simulink model "simulink_group46"  (R2022b)
settings: Solver=FixedStepAuto  StartTime=0.0  StopTime=10  FixedStep=1e-3  RelTol=1e-3  EnableMultiTasking=on
undefined symbols (not defined in the file): A0, A1, D0, D1, D10, D11, D12, D13, D2, D3, D4, D5, D6, D7, D8, D9, PTA0, PTA1, PTA2, PTB2, PTB23, PTB3, PTB9, PTC16, PTC17, PTC2, PTC3, PTC4, PTD0, PTD1, PTD2, PTD3
libraries: frdmk64flib x19, etargetslib x19, dspstat3 x1
settings Model: ExtModeTrigDuration=5  Creator=aliciamorielli  LastModifiedBy=ethan
settings SolverCC: AlgebraicLoopSolver=TrustRegion
settings OptimizationCC: EnhancedBackFolding=on  PassReuseOutputArgsThreshold=0  MaxStackSize=64  OptimizeBlockOrder=speed  DifferentSizesBufferReuse=on  OptimizationCustomize=off
settings DebuggingCC: ParameterTunabilityLossMsg=error  UnconnectedInputMsg=warning  UnconnectedOutputMsg=warning  UnconnectedLineMsg=warning  SFMachineParentedDataDiag=warning
settings HardwareCC: ProdBitPerPointer=32  ProdBitPerSizeT=32  ProdBitPerPtrDiffT=32  ProdLargestAtomicInteger=Long  ProdLargestAtomicFloat=Double  ProdWordSize=32  ProdHWDeviceType=ARM Compatible->ARM Cortex  UseEmbeddedCoderFeatures=off
settings ModelReferenceCC: EnableRefExpFcnMdlSchedulingChecks=on
settings SFSimCC: MATLABDynamicMemAlloc=off
settings RTWCC: Description=Embedded Coder  SystemTargetFile=ert.tlc  HardwareBoard=NXP FRDM-K64F  TLCOptions="-aInlineSetEventsForThisBaseRateFcn=TLC_FALSE -aSuppressMultiTaskScheduler=TLC_FALSE  -aRateBasedStepFcn=0"  TemplateMakefile=ert_default_tmf  Toolchain=GNU Tools for ARM Embedded Processors  DLArmComputeVersion=19.05
settings CodeAppCC: ForceParamTrailComments=on  OperatorAnnotations=on
settings ERTTargetCC: ERTCustomFileBanners=off  SupportContinuousTime=on  SupportNonInlinedSFcns=on  RemoveResetFunc=off  ModelStepFunctionPrototypeControlCompliant=off  ExtModeTransport=4  ExtModeMexFile=sendToCommService

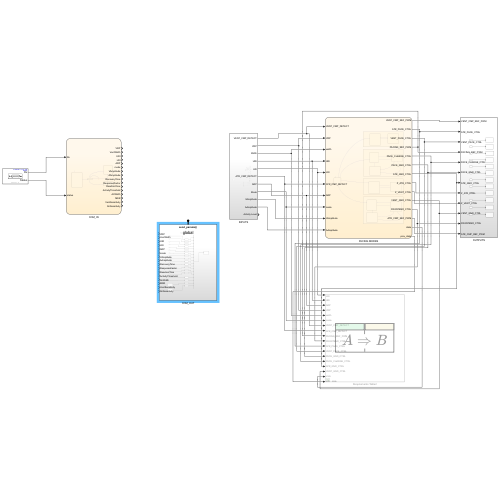
[thumbnail: Simulink's stored preview of the top-level diagram]
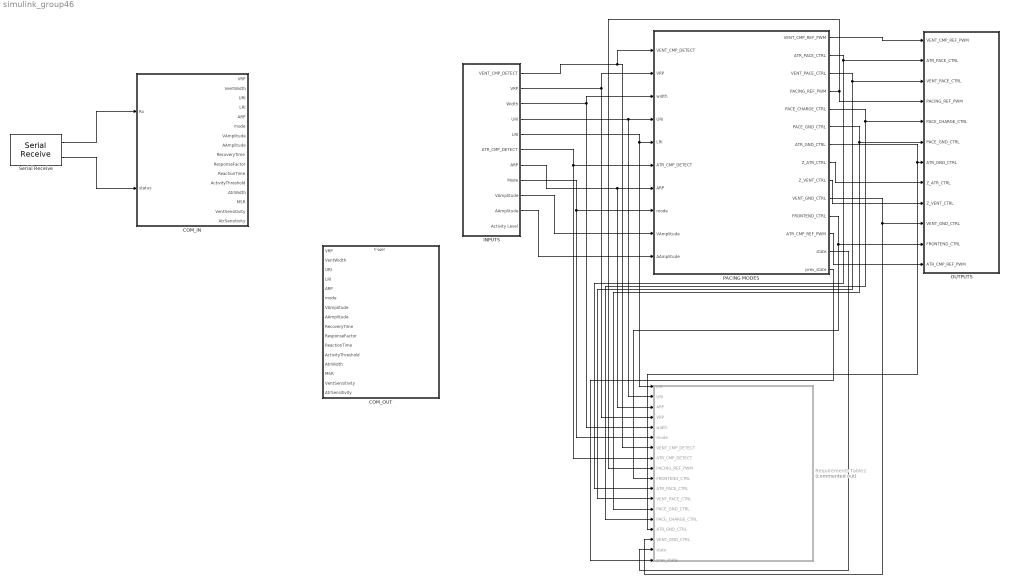
== system simulink_group46 ==
  COM_IN : Stateflow chart  TreatAsAtomicUnit=on
      settings: PortSchema="{\"entries\":[{\"content\":{\"sides\":[{\"content\":{\"connectorIds\":[\"In1\",\"In2\"]},\"type\":\"ConnectorPlacement.EquallySpacedRectSide\",\"uuid\":\"eafe7878-2647-49a4-97cb-41e68478fa40\"},{\"content\":{\"connectorIds\":[\"Out3\",\"Out1\",\"Out5\",\"Out6\",\"Out7\",\"Out2\",\"Out4\",\"Out8\",\"Out9\",\"Out10\",\"Out11\",\"Out12\",\"Out13\",\"Out14\",\"Out15\",\"Out16\"],\"side\":\"RIGHT\"},\"type\":\"ConnectorPlacement.EquallySpacedRectSide\",\"uuid\":\"c0ba33de-ccdc-4037-9e5a-c304987946dd\"},{\"content\":{\"connectorIds\":[],\"side\":\"TOP\"},\"type\":\"ConnectorPlacement.EquallySpacedRectSide\",\"uuid\":\"204d3e33-d140-4353-8067-53c664c1cb64\"}]},\"type\":\"ConnectorPlacement.EquallySpacedConnector\",\"uuid\":\"8b254745-690b-4cb1-aa57-728c67132f0f\"}],\"packageUris\":[\"http://schema.mathworks.com/mf0/Connector/R2020b\"],\"version\":\"1.0\"}"
  COM_OUT : Subsystem  TreatAsAtomicUnit=on
  INPUTS : Subsystem
  OUTPUTS : Subsystem
  PACING MODES : Stateflow chart  TreatAsAtomicUnit=on
      settings: PortSchema="{\"entries\":[{\"content\":{\"sides\":[{\"content\":{\"connectorIds\":[\"In1\",\"In5\",\"In2\",\"In3\",\"In4\",\"In7\",\"In6\",\"In8\",\"In9\",\"In10\"]},\"type\":\"ConnectorPlacement.EquallySpacedRectSide\",\"uuid\":\"24afec03-bc13-4065-9064-27bef3c43f7a\"},{\"content\":{\"connectorIds\":[\"Out11\",\"Out1\",\"Out2\",\"Out3\",\"Out4\",\"Out5\",\"Out6\",\"Out7\",\"Out8\",\"Out9\",\"Out10\",\"Out12\",\"Out13\",\"Out14\"],\"side\":\"RIGHT\"},\"type\":\"ConnectorPlacement.EquallySpacedRectSide\",\"uuid\":\"79d0ee85-df22-4c09-8ba8-cd763efde854\"},{\"content\":{\"connectorIds\":[],\"side\":\"TOP\"},\"type\":\"ConnectorPlacement.EquallySpacedRectSide\",\"uuid\":\"d342e713-b0ae-4b06-a4c2-9648f7d82d61\"},{\"content\":{\"connectorIds\":[],\"side\":\"BOTTOM\"},\"type\":\"ConnectorPlacement.EquallySpacedRectSide\",\"uuid\":\"4b63818c-7bd6-427f-a568-d3913931a17b\"}]},\"type\":\"ConnectorPlacement.EquallySpacedConnector\",\"uuid\":\"408ec0d3-1c59-4342-b3c9-42fd185f3962\"}],\"packageUris\":[\"http://schema.mathworks.com/mf0/Connector/R2020b\"],\"version\":\"1.0\"}"
  Requirements Table2 : Requirements Table  Commented=on  TreatAsAtomicUnit=on
  Serial Receive : frdmk64flib/Serial Receive  SCIModule=0  Baudrate=uint32(9600)  Parity=None  StopBits=1  HardwareFlowControl=None  ByteOrder=LittleEndian  DataType=uint8  DataLength=10  BlockingMode=off  OutputStatus=on  SampleTime=0.1
  wires:
  INPUTS/8(Mode) -> Requirements Table2/6(mode), PACING MODES/8(mode)
  INPUTS/2(VRP) -> Requirements Table2/4(VRP), PACING MODES/5(VRP)
  INPUTS/3(Width) -> Requirements Table2/5(width), PACING MODES/2(width)
  INPUTS/4(URI) -> Requirements Table2/2(URI), PACING MODES/3(URI)
  INPUTS/5(LRI) -> Requirements Table2/1(LRI), PACING MODES/4(LRI)
  INPUTS/6(ATR_CMP_DETECT) -> Requirements Table2/8(ATR_CMP_DETECT), PACING MODES/7(ATR_CMP_DETECT)
  INPUTS/7(ARP) -> Requirements Table2/3(ARP), PACING MODES/6(ARP)
  PACING MODES/11(VENT_CMP_REF_PWM) -> OUTPUTS/1(VENT_CMP_REF_PWM)
  PACING MODES/2(VENT_PACE_CTRL) -> Requirements Table2/12(VENT_PACE_CTRL), OUTPUTS/3(VENT_PACE_CTRL)
  PACING MODES/3(PACING_REF_PWM) -> OUTPUTS/4(PACING_REF_PWM), Requirements Table2/9(PACING_REF_PWM)
  PACING MODES/4(PACE_CHARGE_CTRL) -> Requirements Table2/14(PACE_CHARGE_CTRL), OUTPUTS/5(PACE_CHARGE_CTRL)
  PACING MODES/5(PACE_GND_CTRL) -> Requirements Table2/13(PACE_GND_CTRL), OUTPUTS/6(PACE_GND_CTRL)
  PACING MODES/6(ATR_GND_CTRL) -> Requirements Table2/15(ATR_GND_CTRL), OUTPUTS/7(ATR_GND_CTRL)
  PACING MODES/7(Z_ATR_CTRL) -> OUTPUTS/8(Z_ATR_CTRL)
  PACING MODES/8(Z_VENT_CTRL) -> OUTPUTS/9(Z_VENT_CTRL)
  PACING MODES/9(VENT_GND_CTRL) -> Requirements Table2/16(VENT_GND_CTRL), OUTPUTS/10(VENT_GND_CTRL)
  PACING MODES/10(FRONTEND_CTRL) -> Requirements Table2/10(FRONTEND_CTRL), OUTPUTS/11(FRONTEND_CTRL)
  PACING MODES/12(ATR_CMP_REF_PWM) -> OUTPUTS/12(ATR_CMP_REF_PWM)
  PACING MODES/1(ATR_PACE_CTRL) -> Requirements Table2/11(ATR_PACE_CTRL), OUTPUTS/2(ATR_PACE_CTRL)
  INPUTS/1(VENT_CMP_DETECT) -> Requirements Table2/7(VENT_CMP_DETECT), PACING MODES/1(VENT_CMP_DETECT)
  INPUTS/9(VAmplitude) -> PACING MODES/9(VAmplitude)
  INPUTS/10(AAmplitude) -> PACING MODES/10(AAmplitude)
  PACING MODES/13(state) -> Requirements Table2/17(state)
  PACING MODES/14(prev_state) -> Requirements Table2/18(prev_state)
  Serial Receive/2 -> COM_IN/2(status)
  Serial Receive/1 -> COM_IN/1(Rx)

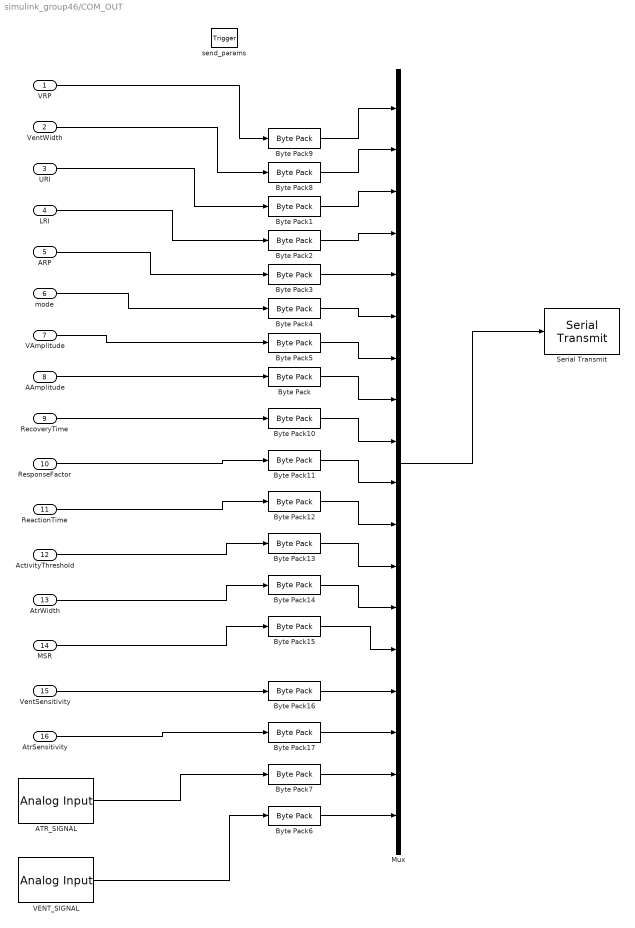
== system simulink_group46/COM_OUT ==
  VRP : Inport
  VentWidth : Inport  Port=2
  URI : Inport  Port=3
  LRI : Inport  Port=4
  ARP : Inport  Port=5
  mode : Inport  Port=6
  VAmplitude : Inport  Port=7
  AAmplitude : Inport  Port=8
  RecoveryTime : Inport  Port=9
  ResponseFactor : Inport  Port=10
  ReactionTime : Inport  Port=11
  ActivityThreshold : Inport  Port=12
  AtrWidth : Inport  Port=13
  MSR : Inport  Port=14
  VentSensitivity : Inport  Port=15
  AtrSensitivity : Inport  Port=16
  send_params : TriggerPort  TriggerType=function-call  IsSimulinkFunction=on  FunctionName=send_params  VariantControl=(inherit)
  ATR_SIGNAL : frdmk64flib/Analog Input  Whichpin=PTB2 (A0)  SampleTime=-1
  Byte Pack{,1..3,5..7,9..17} (16 alike) : etargetslib/Byte Pack  datatypes={'double'}  byteAlign=1
  Byte Pack4 : etargetslib/Byte Pack  datatypes={'int16'}  byteAlign=1
  Byte Pack8 : etargetslib/Byte Pack  datatypes={'int16'}  byteAlign=1
  Mux : Mux  Inputs=18
  Serial Transmit : frdmk64flib/Serial Transmit  SCIModule=0  Baudrate=uint32(9600)  Parity=None  StopBits=1  HardwareFlowControl=None  ByteOrder=LittleEndian  BlockingMode=on  OutputStatus=off
  VENT_SIGNAL : frdmk64flib/Analog Input  Whichpin=PTB3 (A1)  SampleTime=-1
  wires:
  Mux/1 -> Serial Transmit/1
  AAmplitude/1 -> Byte Pack/1
  VAmplitude/1 -> Byte Pack5/1
  mode/1 -> Byte Pack4/1
  ARP/1 -> Byte Pack3/1
  LRI/1 -> Byte Pack2/1
  URI/1 -> Byte Pack1/1
  VentWidth/1 -> Byte Pack8/1
  VRP/1 -> Byte Pack9/1
  ATR_SIGNAL/1 -> Byte Pack7/1
  VENT_SIGNAL/1 -> Byte Pack6/1
  Byte Pack/1 -> Mux/8
  Byte Pack5/1 -> Mux/7
  Byte Pack4/1 -> Mux/6
  Byte Pack3/1 -> Mux/5
  Byte Pack2/1 -> Mux/4
  Byte Pack1/1 -> Mux/3
  Byte Pack8/1 -> Mux/2
  Byte Pack9/1 -> Mux/1
  RecoveryTime/1 -> Byte Pack10/1
  ResponseFactor/1 -> Byte Pack11/1
  ReactionTime/1 -> Byte Pack12/1
  ActivityThreshold/1 -> Byte Pack13/1
  AtrWidth/1 -> Byte Pack14/1
  MSR/1 -> Byte Pack15/1
  Byte Pack10/1 -> Mux/9
  Byte Pack11/1 -> Mux/10
  Byte Pack12/1 -> Mux/11
  Byte Pack13/1 -> Mux/12
  Byte Pack14/1 -> Mux/13
  Byte Pack15/1 -> Mux/14
  VentSensitivity/1 -> Byte Pack16/1
  AtrSensitivity/1 -> Byte Pack17/1
  Byte Pack17/1 -> Mux/16
  Byte Pack16/1 -> Mux/15
  Byte Pack6/1 -> Mux/18
  Byte Pack7/1 -> Mux/17

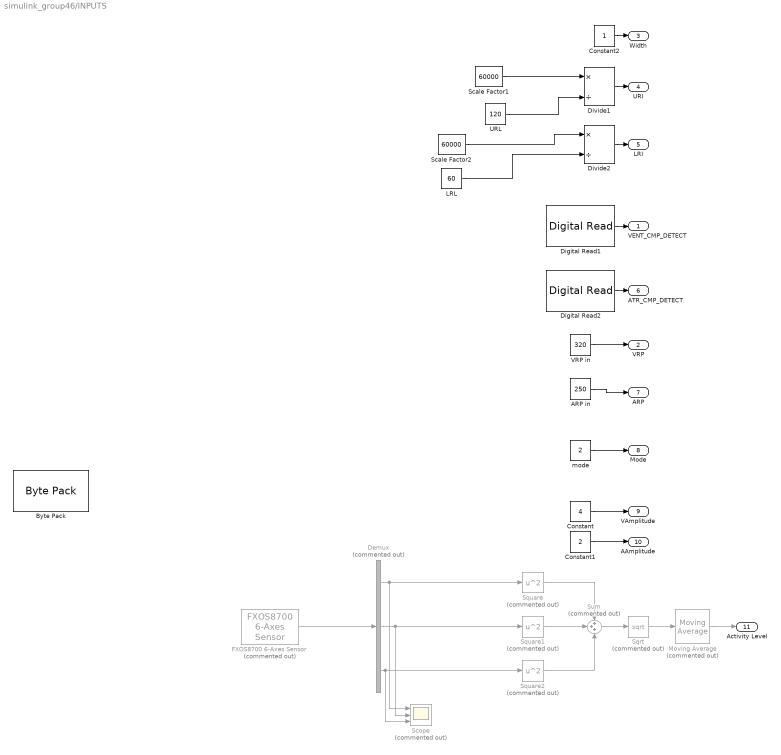
== system simulink_group46/INPUTS ==
  ARP in : Constant  Value=250  OutDataTypeStr=double
  Byte Pack : etargetslib/Byte Pack  datatypes={'double'}  byteAlign=1
  Constant : Constant  Value=4  OutMin=0  OutMax=5  OutDataTypeStr=double
  Constant1 : Constant  Value=2  OutMin=0  OutMax=5  OutDataTypeStr=double
  Constant2 : Constant  OutDataTypeStr=int16
  Demux : Demux  Commented=on  Outputs=3
  Digital Read1 : frdmk64flib/Digital Read  Whichpin=PTC17 (D1)  SampleTime=-1
  Digital Read2 : frdmk64flib/Digital Read  Whichpin=PTC16 (D0)  SampleTime=-1
  Divide1 : Product  Inputs=*/  OutDataTypeStr=double
  Divide2 : Product  Inputs=*/  OutDataTypeStr=double
  FXOS8700 6-Axes Sensor : frdmk64flib/FXOS8700 6-Axes Sensor  Commented=on  Activesensor=Accelerometer only  ODR=800Hz  HybridODR=400Hz  Accelfullrange=-4g to +4g  SampleTime=-1
  LRL : Constant  Value=60  OutDataTypeStr=int16
  Moving Average : dspstat3/Moving Average  Commented=on  Method=Sliding window  ForgettingFactorPort=off  SpecifyWindowLength=on  WindowLength=4  OverlapLength=3  AllowArbitraryInputLength=off  ForgettingFactor=0.9  SimulateUsing=Code generation
  Scale Factor1 : Constant  Value=60000  OutDataTypeStr=int64
  Scale Factor2 : Constant  Value=60000  OutDataTypeStr=int64
  Scope : Scope  Commented=on  NumInputPorts=3
  Sqrt : Sqrt  Commented=on
  Square : Math  Commented=on  Operator=square
  Square1 : Math  Commented=on  Operator=square
  Square2 : Math  Commented=on  Operator=square
  Sum : Sum  Commented=on  Inputs=+++
  URL : Constant  Value=120  OutDataTypeStr=int16
  VRP in : Constant  Value=320  OutDataTypeStr=double
  mode : Constant  Value=2  OutDataTypeStr=int16
  VENT_CMP_DETECT : Outport  OutDataTypeStr=boolean
  VRP : Outport  Port=2  OutDataTypeStr=double
  Width : Outport  Port=3  OutDataTypeStr=int16
  URI : Outport  Port=4  OutDataTypeStr=double
  LRI : Outport  Port=5  OutDataTypeStr=double
  ATR_CMP_DETECT : Outport  Port=6  OutDataTypeStr=boolean
  ARP : Outport  Port=7  OutDataTypeStr=double
  Mode : Outport  Port=8  OutDataTypeStr=int16
  VAmplitude : Outport  Port=9  OutDataTypeStr=double
  AAmplitude : Outport  Port=10  OutDataTypeStr=double
  Activity Level : Outport  Port=11
  wires:
  Scale Factor1/1 -> Divide1/1
  URL/1 -> Divide1/2
  Divide1/1 -> URI/1
  Scale Factor2/1 -> Divide2/1
  Constant2/1 -> Width/1
  LRL/1 -> Divide2/2
  Digital Read1/1 -> VENT_CMP_DETECT/1
  VRP in/1 -> VRP/1
  Divide2/1 -> LRI/1
  ARP in/1 -> ARP/1
  Digital Read2/1 -> ATR_CMP_DETECT/1
  mode/1 -> Mode/1
  Sum/1 -> Sqrt/1
  Sqrt/1 -> Moving Average/1
  Square/1 -> Sum/1
  Square1/1 -> Sum/2
  Square2/1 -> Sum/3
  Demux/2 -> Scope/2, Square1/1
  Demux/3 -> Square2/1, Scope/3
  Demux/1 -> Scope/1, Square/1
  Moving Average/1 -> Activity Level/1
  Constant/1 -> VAmplitude/1
  Constant1/1 -> AAmplitude/1
  FXOS8700 6-Axes Sensor/1 -> Demux/1

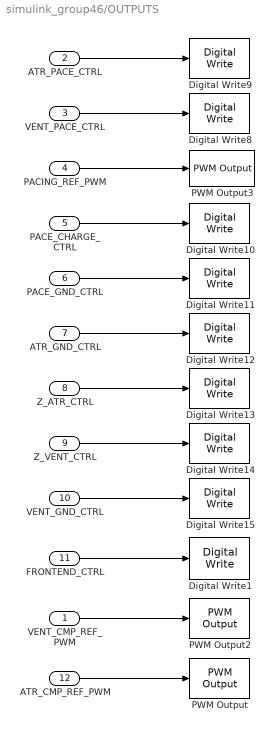
== system simulink_group46/OUTPUTS ==
  VENT_CMP_REF_PWM : Inport  OutDataTypeStr=double
  ATR_PACE_CTRL : Inport  Port=2  OutDataTypeStr=boolean
  VENT_PACE_CTRL : Inport  Port=3  OutDataTypeStr=boolean
  PACING_REF_PWM : Inport  Port=4  OutDataTypeStr=double
  PACE_CHARGE_CTRL : Inport  Port=5  OutDataTypeStr=boolean
  PACE_GND_CTRL : Inport  Port=6  OutDataTypeStr=boolean
  ATR_GND_CTRL : Inport  Port=7  OutDataTypeStr=boolean
  Z_ATR_CTRL : Inport  Port=8  OutDataTypeStr=boolean
  Z_VENT_CTRL : Inport  Port=9  OutDataTypeStr=boolean
  VENT_GND_CTRL : Inport  Port=10  OutDataTypeStr=boolean
  FRONTEND_CTRL : Inport  Port=11  OutDataTypeStr=boolean
  ATR_CMP_REF_PWM : Inport  Port=12  OutDataTypeStr=int16
  Digital Write1 : frdmk64flib/Digital Write  Whichpin=PTD1 (D13)
  Digital Write10 : frdmk64flib/Digital Write  Whichpin=PTB9 (D2)
  Digital Write11 : frdmk64flib/Digital Write  Whichpin=PTD0 (D10)
  Digital Write12 : frdmk64flib/Digital Write  Whichpin=PTD2 (D11)
  Digital Write13 : frdmk64flib/Digital Write  Whichpin=PTB23 (D4)
  Digital Write14 : frdmk64flib/Digital Write  Whichpin=PTC3 (D7)
  Digital Write15 : frdmk64flib/Digital Write  Whichpin=PTD3 (D12)
  Digital Write8 : frdmk64flib/Digital Write  Whichpin=PTC4 (D9)
  Digital Write9 : frdmk64flib/Digital Write  Whichpin=PTA0 (D8)
  PWM Output : frdmk64flib/PWM Output  Whichpin=PTC2 (D6)  InitialFrequency=2000  InitialDutyCycle=53
  PWM Output2 : frdmk64flib/PWM Output  Whichpin=PTA1 (D3)  InitialFrequency=2000  InitialDutyCycle=53
  PWM Output3 : frdmk64flib/PWM Output  Whichpin=PTA2 (D5)  InitialFrequency=2000  InitialDutyCycle=40
  wires:
  Z_ATR_CTRL/1 -> Digital Write13/1
  Z_VENT_CTRL/1 -> Digital Write14/1
  FRONTEND_CTRL/1 -> Digital Write1/1
  PACE_CHARGE_CTRL/1 -> Digital Write10/1
  VENT_PACE_CTRL/1 -> Digital Write8/1
  ATR_CMP_REF_PWM/1 -> PWM Output/1
  VENT_CMP_REF_PWM/1 -> PWM Output2/1
  ATR_GND_CTRL/1 -> Digital Write12/1
  ATR_PACE_CTRL/1 -> Digital Write9/1
  VENT_GND_CTRL/1 -> Digital Write15/1
  PACE_GND_CTRL/1 -> Digital Write11/1
  PACING_REF_PWM/1 -> PWM Output3/1

== stateflow chart simulink_group46/COM_IN ==
  state SET_PARAM
    entry:
  state INITIAL
    entry:
    VentWidth = 1;
    AtrWidth = 1;
    URI = 500;
    LRI = 1000;
    VRP = 320;
    ARP = 250;
    mode = 0;
    VAmplitude = 4;
    AAmplitude = 4;
    ReactionTime = 30;
    ResponseFactor = 8;
    RecoveryTime = 300;
    ActivityThreshold = 4;
    MSR = 120;
    VentSensitivity = 3;
    AtrSensitivity = 3;
  state STANDBY
  state ECHO_PARAM
    entry:
    send_params();
  (default) -> INITIAL
  SET_PARAM -> STANDBY
  (junction 18) -> SET_PARAM [order 1] : [Rx(2) == hex2dec('22')]
  (junction 14) -> STANDBY [order 2]
  STANDBY -> (junction 14) : [status == 0]
  (junction 14) -> (junction 18) [order 1] : [Rx(1) == hex2dec('16')]
  INITIAL -> STANDBY
  (junction 18) -> ECHO_PARAM [order 2] : [Rx(2) == hex2dec('33')]
  ECHO_PARAM -> STANDBY
  data: Rx input uint8; status input uint8; VentWidth output int16; mode output int16; VRP output double; VAmplitude output double; URI output double; LRI output double; ARP output double; AAmplitude output double; RecoveryTime output double; ResponseFactor output double; ReactionTime output double; ActivityThreshold output int16; AtrWidth output int16; MSR output double; VentSensitivity output double; AtrSensitivity output double

== stateflow chart simulink_group46/Requirements Table2 ==
  (default) -> (junction 1073752909)
  (junction 1073752909) -> (junction 1073752910) : {
      | % SF_REQ_REV_07
      | }
  (junction 1073752910) -> (junction 1073752912) : {
      | % HEADER_ASSIGNMENTS
      |
      | }
  (junction 1073752912) -> (junction 1073752914) : {
      | % START_A_4
      | }
  (junction 1073752914) -> (junction 1073752916) : {
      | }
  (junction 1073752916) -> (junction 1073752918) : {
      | reqtable_assumption((LRI <= 1200 && LRI >= (60000/90)), 4);
      | }
  (junction 1073752918) -> (junction 1073752920) : {
      | }
  (junction 1073752920) -> (junction 1073752922) : {
      | % END_A_4
      | }
  (junction 1073752922) -> (junction 1073752924) : {
      | % START_A_7
      | }
  (junction 1073752924) -> (junction 1073752926) : {
      | }
  (junction 1073752926) -> (junction 1073752928) : {
      | reqtable_assumption((URI <= 1200 && URI >= (60000/175)), 7);
      | }
  (junction 1073752928) -> (junction 1073752930) : {
      | }
  (junction 1073752930) -> (junction 1073752932) : {
      | % END_A_7
      | }
  (junction 1073752932) -> (junction 1073752934) : {
      | % START_A_10
      | }
  (junction 1073752934) -> (junction 1073752936) : {
      | }
  (junction 1073752936) -> (junction 1073752938) : {
      | reqtable_assumption((PACING_REF_PWM <= 64), 10);
      | }
  (junction 1073752938) -> (junction 1073752940) : {
      | }
  (junction 1073752940) -> (junction 1073752942) : {
      | % END_A_10
      | }
  (junction 1073752942) -> (junction 1073752944) : {
      | % START_A_13
      | }
  (junction 1073752944) -> (junction 1073752946) : {
      | }
  (junction 1073752946) -> (junction 1073752948) : {
      | reqtable_assumption((width == 1), 13);
      | }
  (junction 1073752948) -> (junction 1073752950) : {
      | }
  (junction 1073752950) -> (junction 1073752952) : {
      | % END_A_13
      | }
  (junction 1073752952) -> (junction 1073752954) : {
      | % START_A_16
      | }
  (junction 1073752954) -> (junction 1073752956) : {
      | }
  (junction 1073752956) -> (junction 1073752958) : {
      | reqtable_assumption((VRP >= 150 && VRP <= 500), 16);
      | }
  (junction 1073752958) -> (junction 1073752960) : {
      | }
  (junction 1073752960) -> (junction 1073752962) : {
      | % END_A_16
      | }
  (junction 1073752962) -> (junction 1073752964) : {
      | % START_A_19
      | }
  (junction 1073752964) -> (junction 1073752966) : {
      | }
  (junction 1073752966) -> (junction 1073752968) : {
      | reqtable_assumption((ARP >= 150 && ARP <= 500), 19);
      | }
  (junction 1073752968) -> (junction 1073752970) : {
      | }
  (junction 1073752970) -> (junction 1073752972) : {
      | % END_A_19
      | }
  (junction 1073752972) -> (junction 1073752974) : {
      | % START_A_22
      | }
  (junction 1073752974) -> (junction 1073752976) : {
      | }
  (junction 1073752976) -> (junction 1073752978) : {
      | reqtable_assumption((mode >= 1 && mode <= 4), 22);
      | }
  (junction 1073752978) -> (junction 1073752980) : {
      | }
  (junction 1073752980) -> (junction 1073752982) : {
      | % END_A_22
      | }
  (junction 1073752982) -> (junction 1073752984) : {
      | % START_R_1
      | }
  (junction 1073752984) -> (junction 1073752986) : {
      | }
  (junction 1073752986) -> (junction 1073752988)
  (junction 1073752988) -> (junction 1073752990) [order 1] : [(((mode) == (2))) && (((FRONTEND_CTRL) == (true))) && (((PACE_CHARGE_CTRL) == (true))) && (((PACE_GND_CTRL) == (true))) && (((ATR_CMP_DETECT) == (true)) || ((ATR_CMP_DETECT) == (false)))]
  (junction 1073752988) -> (junction 1073753032) [order 2]
  (junction 1073752990) -> (junction 1073752992) : {
      | reqtable_postcondition((((ATR_PACE_CTRL) == (false))) && (((ATR_GND_CTRL) == (true)) || ((ATR_GND_CTRL) == (false))), 'R:1');
      |
      |
      | }
  (junction 1073752992) -> (junction 1073752994) : {
      | }
  (junction 1073752994) -> (junction 1073752996) : {
      | % START_R_79
      | }
  (junction 1073752996) -> (junction 1073752998) : {
      | }
  (junction 1073752998) -> (junction 1073753000)
  (junction 1073753000) -> (junction 1073753002) [order 1] : [(((VENT_CMP_DETECT) == (false))) && (((prev_state) == (2)))]
  (junction 1073753000) -> (junction 1073753008) [order 2]
  (junction 1073753002) -> (junction 1073753004) : {
      | reqtable_postcondition((((VENT_PACE_CTRL) == (true))) && (((VENT_GND_CTRL) == (true))) && (((state) == (3))), 'R:1.1');
      |
      |
      | }
  (junction 1073753004) -> (junction 1073753006) : {
      | }
  (junction 1073753006) -> (junction 1073753008)
  (junction 1073753008) -> (junction 1073753010)
  (junction 1073753010) -> (junction 1073753012) : {
      | % END_R_79
      | }
  (junction 1073753012) -> (junction 1073753014) : {
      | % START_R_82
      | }
  (junction 1073753014) -> (junction 1073753016) : {
      | }
  (junction 1073753016) -> (junction 1073753018)
  (junction 1073753018) -> (junction 1073753020) [order 1] : [(((VENT_CMP_DETECT) == (true))) && (((prev_state) == (1)))]
  (junction 1073753018) -> (junction 1073753026) [order 2]
  (junction 1073753020) -> (junction 1073753022) : {
      | reqtable_postcondition((((VENT_PACE_CTRL) == (false))) && (((VENT_GND_CTRL) == (false))) && (((state) == (1))), 'R:1.2');
      |
      |
      | }
  (junction 1073753022) -> (junction 1073753024) : {
      | }
  (junction 1073753024) -> (junction 1073753026)
  (junction 1073753026) -> (junction 1073753028)
  (junction 1073753028) -> (junction 1073753030) : {
      | % END_R_82
      | }
  (junction 1073753030) -> (junction 1073753032)
  (junction 1073753032) -> (junction 1073753034)
  (junction 1073753034) -> (junction 1073753036) : {
      | % END_R_1
      | }
  (junction 1073753036) -> (junction 1073753038) : {
      | % START_R_28
      | }
  (junction 1073753038) -> (junction 1073753040) : {
      | }
  (junction 1073753040) -> (junction 1073753042)
  (junction 1073753042) -> (junction 1073753044) [order 1] : [(((mode) == (1)) || ((mode) == (2))) && (((FRONTEND_CTRL) == (false))) && (((PACE_CHARGE_CTRL) == (false))) && (((PACE_GND_CTRL) == (true))) && (((VENT_CMP_DETECT) == (false))) && (((ATR_CMP_DETECT) == (true)) || ((ATR_CMP_DETECT) == (false))) && (((prev_state) == (1)))]
  (junction 1073753042) -> (junction 1073753050) [order 2]
  (junction 1073753044) -> (junction 1073753046) : {
      | reqtable_postcondition((((VENT_PACE_CTRL) == (true))) && (((ATR_PACE_CTRL) == (false))) && (((VENT_GND_CTRL) == (false))) && (((ATR_GND_CTRL) == (true)) || ((ATR_GND_CTRL) == (false))) && (((state) == (1))), 'R:2');
      |
      |
      | }
  (junction 1073753046) -> (junction 1073753048) : {
      | }
  (junction 1073753048) -> (junction 1073753050)
  (junction 1073753050) -> (junction 1073753052)
  (junction 1073753052) -> (junction 1073753054) : {
      | % END_R_28
      | }
  (junction 1073753054) -> (junction 1073753056) : {
      | % START_R_46
      | }
  (junction 1073753056) -> (junction 1073753058) : {
      | }
  (junction 1073753058) -> (junction 1073753060) : {
      |
      |
      | }
  (junction 1073753060) -> (junction 1073753062) : {
      | }
  (junction 1073753062) -> (junction 1073753064) : {
      | % START_R_61
      | }
  (junction 1073753064) -> (junction 1073753066) : {
      | }
  (junction 1073753066) -> (junction 1073753068)
  (junction 1073753068) -> (junction 1073753070) [order 1] : [(((mode) == (1))) && (((FRONTEND_CTRL) == (false))) && (((PACE_CHARGE_CTRL) == (true))) && (((PACE_GND_CTRL) == (true))) && (((VENT_CMP_DETECT) == (true)) || ((VENT_CMP_DETECT) == (false))) && (((ATR_CMP_DETECT) == (true)) || ((ATR_CMP_DETECT) == (false))) && (((prev_state) == (2)))]
  (junction 1073753068) -> (junction 1073753076) [order 2]
  (junction 1073753070) -> (junction 1073753072) : {
      | reqtable_postcondition((((VENT_PACE_CTRL) == (false))) && (((ATR_PACE_CTRL) == (true)) || ((ATR_PACE_CTRL) == (false))) && (((VENT_GND_CTRL) == (true))) && (((ATR_GND_CTRL) == (true)) || ((ATR_GND_CTRL) == (false))) && (((state) == (2))), 'R:3.1');
      |
      |
      | }
  (junction 1073753072) -> (junction 1073753074) : {
      | }
  (junction 1073753074) -> (junction 1073753076)
  (junction 1073753076) -> (junction 1073753078)
  (junction 1073753078) -> (junction 1073753080) : {
      | % END_R_61
      | }
  (junction 1073753080) -> (junction 1073753082) : {
      | % START_R_64
      | }
  (junction 1073753082) -> (junction 1073753084) : {
      | }
  (junction 1073753084) -> (junction 1073753086)
  (junction 1073753086) -> (junction 1073753088) [order 1] : [(((mode) == (2))) && (((FRONTEND_CTRL) == (true)) || ((FRONTEND_CTRL) == (false))) && (((PACE_CHARGE_CTRL) == (true))) && (((PACE_GND_CTRL) == (true))) && (((VENT_CMP_DETECT) == (true)) || ((VENT_CMP_DETECT) == (false))) && (((ATR_CMP_DETECT) == (true)) || ((ATR_CMP_DETECT) == (false))) && (((prev_state) == (1)))]
  (junction 1073753086) -> (junction 1073753094) [order 2]
  (junction 1073753088) -> (junction 1073753090) : {
      | reqtable_postcondition((((VENT_PACE_CTRL) == (false))) && (((ATR_PACE_CTRL) == (true)) || ((ATR_PACE_CTRL) == (false))) && (((VENT_GND_CTRL) == (true))) && (((ATR_GND_CTRL) == (true)) || ((ATR_GND_CTRL) == (false))) && (((state) == (2))), 'R:3.2');
      |
      |
      | }
  (junction 1073753090) -> (junction 1073753092) : {
      | }
  (junction 1073753092) -> (junction 1073753094)
  (junction 1073753094) -> (junction 1073753096)
  (junction 1073753096) -> (junction 1073753098) : {
      | % END_R_64
      | }
  (junction 1073753098) -> (junction 1073753100) : {
      | % END_R_46
      | }
  (junction 1073753100) -> (junction 1073753102) : {
      | % START_R_31
      | }
  (junction 1073753102) -> (junction 1073753104) : {
      | }
  (junction 1073753104) -> (junction 1073753106)
  (junction 1073753106) -> (junction 1073753108) [order 1] : [(((mode) == (4))) && (((FRONTEND_CTRL) == (true))) && (((PACE_CHARGE_CTRL) == (true))) && (((PACE_GND_CTRL) == (true))) && (((VENT_CMP_DETECT) == (true)) || ((VENT_CMP_DETECT) == (false)))]
  (junction 1073753106) -> (junction 1073753150) [order 2]
  (junction 1073753108) -> (junction 1073753110) : {
      | reqtable_postcondition((((VENT_PACE_CTRL) == (false))) && (((VENT_GND_CTRL) == (true)) || ((VENT_GND_CTRL) == (false))), 'R:4');
      |
      |
      | }
  (junction 1073753110) -> (junction 1073753112) : {
      | }
  (junction 1073753112) -> (junction 1073753114) : {
      | % START_R_85
      | }
  (junction 1073753114) -> (junction 1073753116) : {
      | }
  (junction 1073753116) -> (junction 1073753118)
  (junction 1073753118) -> (junction 1073753120) [order 1] : [(((ATR_CMP_DETECT) == (false))) && (((prev_state) == (2)))]
  (junction 1073753118) -> (junction 1073753126) [order 2]
  (junction 1073753120) -> (junction 1073753122) : {
      | reqtable_postcondition((((ATR_PACE_CTRL) == (true))) && (((ATR_GND_CTRL) == (true))) && (((state) == (3))), 'R:4.1');
      |
      |
      | }
  (junction 1073753122) -> (junction 1073753124) : {
      | }
  (junction 1073753124) -> (junction 1073753126)
  (junction 1073753126) -> (junction 1073753128)
  (junction 1073753128) -> (junction 1073753130) : {
      | % END_R_85
      | }
  (junction 1073753130) -> (junction 1073753132) : {
      | % START_R_88
      | }
  (junction 1073753132) -> (junction 1073753134) : {
      | }
  (junction 1073753134) -> (junction 1073753136)
  (junction 1073753136) -> (junction 1073753138) [order 1] : [(((ATR_CMP_DETECT) == (true))) && (((prev_state) == (1)))]
  (junction 1073753136) -> (junction 1073753144) [order 2]
  (junction 1073753138) -> (junction 1073753140) : {
      | reqtable_postcondition((((ATR_PACE_CTRL) == (false))) && (((ATR_GND_CTRL) == (false))) && (((state) == (1))), 'R:4.2');
      |
      |
      | }
  (junction 1073753140) -> (junction 1073753142) : {
      | }
  (junction 1073753142) -> (junction 1073753144)
  (junction 1073753144) -> (junction 1073753146)
  (junction 1073753146) -> (junction 1073753148) : {
      | % END_R_88
      | }
  (junction 1073753148) -> (junction 1073753150)
  (junction 1073753150) -> (junction 1073753152)
  (junction 1073753152) -> (junction 1073753154) : {
      | % END_R_31
      | }
  (junction 1073753154) -> (junction 1073753156) : {
      | % START_R_37
      | }
  (junction 1073753156) -> (junction 1073753158) : {
      | }
  (junction 1073753158) -> (junction 1073753160)
  (junction 1073753160) -> (junction 1073753162) [order 1] : [(((mode) == (3)) || ((mode) == (4))) && (((FRONTEND_CTRL) == (false))) && (((PACE_CHARGE_CTRL) == (false))) && (((PACE_GND_CTRL) == (true))) && (((VENT_CMP_DETECT) == (true)) || ((VENT_CMP_DETECT) == (false))) && (((ATR_CMP_DETECT) == (false))) && (((prev_state) == (1)))]
  (junction 1073753160) -> (junction 1073753168) [order 2]
  (junction 1073753162) -> (junction 1073753164) : {
      | reqtable_postcondition((((VENT_PACE_CTRL) == (false))) && (((ATR_PACE_CTRL) == (true))) && (((VENT_GND_CTRL) == (true)) || ((VENT_GND_CTRL) == (false))) && (((ATR_GND_CTRL) == (false))) && (((state) == (1))), 'R:5');
      |
      |
      | }
  (junction 1073753164) -> (junction 1073753166) : {
      | }
  (junction 1073753166) -> (junction 1073753168)
  (junction 1073753168) -> (junction 1073753170)
  (junction 1073753170) -> (junction 1073753172) : {
      | % END_R_37
      | }
  (junction 1073753172) -> (junction 1073753174) : {
      | % START_R_55
      | }
  (junction 1073753174) -> (junction 1073753176) : {
      | }
  (junction 1073753176) -> (junction 1073753178) : {
      |
      |
      | }
  (junction 1073753178) -> (junction 1073753180) : {
      | }
  (junction 1073753180) -> (junction 1073753182) : {
      | % START_R_67
      | }
  (junction 1073753182) -> (junction 1073753184) : {
      | }
  (junction 1073753184) -> (junction 1073753186)
  (junction 1073753186) -> (junction 1073753188) [order 1] : [(((mode) == (3))) && (((FRONTEND_CTRL) == (false))) && (((PACE_CHARGE_CTRL) == (true))) && (((PACE_GND_CTRL) == (true))) && (((VENT_CMP_DETECT) == (true)) || ((VENT_CMP_DETECT) == (false))) && (((ATR_CMP_DETECT) == (true)) || ((ATR_CMP_DETECT) == (false))) && (((prev_state) == (2)))]
  (junction 1073753186) -> (junction 1073753194) [order 2]
  (junction 1073753188) -> (junction 1073753190) : {
      | reqtable_postcondition((((VENT_PACE_CTRL) == (true)) || ((VENT_PACE_CTRL) == (false))) && (((ATR_PACE_CTRL) == (false))) && (((VENT_GND_CTRL) == (true)) || ((VENT_GND_CTRL) == (false))) && (((ATR_GND_CTRL) == (true))) && (((state) == (2))), 'R:6.1');
      |
      |
      | }
  (junction 1073753190) -> (junction 1073753192) : {
      | }
  (junction 1073753192) -> (junction 1073753194)
  (junction 1073753194) -> (junction 1073753196)
  (junction 1073753196) -> (junction 1073753198) : {
      | % END_R_67
      | }
  (junction 1073753198) -> (junction 1073753200) : {
      | % START_R_70
      | }
  (junction 1073753200) -> (junction 1073753202) : {
      | }
  (junction 1073753202) -> (junction 1073753204)
  (junction 1073753204) -> (junction 1073753206) [order 1] : [(((mode) == (4))) && (((FRONTEND_CTRL) == (true)) || ((FRONTEND_CTRL) == (false))) && (((PACE_CHARGE_CTRL) == (true))) && (((PACE_GND_CTRL) == (true))) && (((VENT_CMP_DETECT) == (true)) || ((VENT_CMP_DETECT) == (false))) && (((ATR_CMP_DETECT) == (true)) || ((ATR_CMP_DETECT) == (false))) && (((prev_state) == (1)))]
  (junction 1073753204) -> (junction 1073753212) [order 2]
  (junction 1073753206) -> (junction 1073753208) : {
      | reqtable_postcondition((((VENT_PACE_CTRL) == (true)) || ((VENT_PACE_CTRL) == (false))) && (((ATR_PACE_CTRL) == (false))) && (((VENT_GND_CTRL) == (true)) || ((VENT_GND_CTRL) == (false))) && (((ATR_GND_CTRL) == (true))) && (((state) == (2))), 'R:6.2');
      |
      |
      | }
  (junction 1073753208) -> (junction 1073753210) : {
      | }
  (junction 1073753210) -> (junction 1073753212)
  (junction 1073753212) -> (junction 1073753214)
  (junction 1073753214) -> (junction 1073753216) : {
      | % END_R_70
      | }
  (junction 1073753216) -> (junction 1073753218) : {
      | % END_R_55
      | }
  (junction 1073753218) -> (junction 1073753220) : {
      | % START_R_76
      | }
  (junction 1073753220) -> (junction 1073753222) : {
      | }
  (junction 1073753222) -> (junction 1073753224)
  (junction 1073753224) -> (junction 1073753226) [order 1] : [(((mode) == (1)) || ((mode) == (2)) || ((mode) == (3)) || ((mode) == (4))) && (((prev_state) >= (0) && (prev_state) <= (3)))]
  (junction 1073753224) -> (junction 1073753232) [order 2]
  (junction 1073753226) -> (junction 1073753228) : {
      | reqtable_postcondition((((VENT_PACE_CTRL) == (true)) || ((VENT_PACE_CTRL) == (false))) && (((ATR_PACE_CTRL) == (true)) || ((ATR_PACE_CTRL) == (false))) && (((VENT_GND_CTRL) == (true)) || ((VENT_GND_CTRL) == (false))) && (((ATR_GND_CTRL) == (true)) || ((ATR_GND_CTRL) == (false))) && (((state) >= (0) && (state) <= (3))), 'R:7');
      |
      |
      | }
  (junction 1073753228) -> (junction 1073753230) : {
      | }
  (junction 1073753230) -> (junction 1073753232)
  (junction 1073753232) -> (junction 1073753234)
  (junction 1073753234) -> (junction 1073753236) : {
      | % END_R_76
      | }
  data: LRI input double; URI input double; ARP input double; VRP input double; width input int16; mode input int16; VENT_CMP_DETECT input boolean; ATR_CMP_DETECT input boolean; PACING_REF_PWM input double; FRONTEND_CTRL input boolean; ATR_PACE_CTRL input boolean; VENT_PACE_CTRL input boolean; PACE_GND_CTRL input boolean; PACE_CHARGE_CTRL input boolean; ATR_GND_CTRL input boolean; VENT_GND_CTRL input boolean; state input int16; prev_state input int16

== stateflow chart simulink_group46/PACING MODES ==
  state VOO [group]
    state Charge_C22_VOO
      entry:
      ATR_PACE_CTRL = false;
      VENT_PACE_CTRL = false;
      PACING_REF_PWM = VAmplitude/5*100;
      PACE_CHARGE_CTRL = true;
      %Discharge C21
      PACE_GND_CTRL = true;
      VENT_PACE_CTRL = false;
      Z_ATR_CTRL = false;
      Z_VENT_CTRL = false;
      ATR_PACE_CTRL = false;
      ATR_GND_CTRL = false;
      VENT_GND_CTRL = true;
      state = 1;
      prev_state = 2;
    state Discharge_C22_VENT_VOO
      entry:
      PACE_CHARGE_CTRL = false;
      PACE_GND_CTRL = true;
      ATR_PACE_CTRL = false;
      ATR_GND_CTRL = false;
      Z_ATR_CTRL = false;
      Z_VENT_CTRL = false;
      VENT_GND_CTRL = false;
      VENT_PACE_CTRL = true;
      state = 2;
      prev_state = 1;
      %
    Discharge_C22_VENT_VOO -> Charge_C22_VOO : [after(LRI,msec)]
    Charge_C22_VOO -> Discharge_C22_VENT_VOO : [after(width,msec)]
  state VVI [group]
    state Wait_VVI
      entry:
      VENT_CMP_REF_PWM = 70;
      FRONTEND_CTRL = false;
      %Discharge C21
      PACE_GND_CTRL = true;
      VENT_PACE_CTRL = false;
      Z_ATR_CTRL = false;
      Z_VENT_CTRL = false;
      ATR_PACE_CTRL = false;
      ATR_GND_CTRL = false;
      VENT_GND_CTRL = true;
      PACE_CHARGE_CTRL = true;
      state = 1;
    state Sensing_Charge_C22_VVI
      entry:
      FRONTEND_CTRL = true;
      %Charge C22
      ATR_PACE_CTRL = false;
      VENT_PACE_CTRL = false;
      PACING_REF_PWM = (VAmplitude/5)*100;
      PACE_CHARGE_CTRL = true;
      state = 2;
      prev_state = 1;
    state Discharge_C22_VENT_VVI
      entry:
      PACE_CHARGE_CTRL = false;
      PACE_GND_CTRL = true;
      ATR_PACE_CTRL = false;
      ATR_GND_CTRL = false;
      Z_ATR_CTRL = false;
      Z_VENT_CTRL = false;
      VENT_GND_CTRL = false;
      VENT_PACE_CTRL = true;
      state = 3;
      prev_state = 2;
    Wait_VVI -> Sensing_Charge_C22_VVI : [after(VRP, msec)]
    Sensing_Charge_C22_VVI -> Wait_VVI [order 1] : [VENT_CMP_DETECT == true]{natural = true}
    Sensing_Charge_C22_VVI -> Discharge_C22_VENT_VVI [order 2] : [after(LRI-VRP,msec) && natural == true]{natural = false}
    Sensing_Charge_C22_VVI -> Discharge_C22_VENT_VVI [order 3] : [after(LRI-VRP-width,msec) && natural == false]
    Discharge_C22_VENT_VVI -> Wait_VVI : [after(width,msec)]
  state Mode_Selector
    entry:
    state = 0;
    prev_state = 0;
    natural = false;
    %Mode 1: VOO
    %Mode 2: VVI
    %Mode 3: AOO
    %Mode 4: AAI
  state AOO [group]
    state Charge_C22_AOO
      entry:
      ATR_PACE_CTRL = false;
      VENT_PACE_CTRL = false;
      PACING_REF_PWM = (AAmplitude/5)*100;
      PACE_CHARGE_CTRL = true;
      %Discharge C21
      PACE_GND_CTRL = true;
      VENT_PACE_CTRL = false;
      Z_ATR_CTRL = false;
      Z_VENT_CTRL = false;
      ATR_PACE_CTRL = false;
      VENT_GND_CTRL = false;
      ATR_GND_CTRL = true;
      state = 1;
      prev_state = 2;
      %
    state Discharge_C22_ATR_AOO
      entry:
      PACE_CHARGE_CTRL = false;
      PACE_GND_CTRL = true;
      VENT_PACE_CTRL = false;
      ATR_GND_CTRL = false;
      Z_ATR_CTRL = false;
      Z_VENT_CTRL = false;
      VENT_GND_CTRL = false;
      ATR_PACE_CTRL = true;
      state = 2;
      prev_state = 1;
      %
    Charge_C22_AOO -> Discharge_C22_ATR_AOO : [after(LRI,msec)]
    Discharge_C22_ATR_AOO -> Charge_C22_AOO : after(width,msec)
  state AAI [group]
    state Wait_AAI
      entry:
      ATR_CMP_REF_PWM = 53;
      FRONTEND_CTRL = false;
      %Discharge C21
      PACE_GND_CTRL = true;
      VENT_PACE_CTRL = false;
      Z_ATR_CTRL = false;
      Z_VENT_CTRL = false;
      ATR_PACE_CTRL = false;
      VENT_GND_CTRL = false;
      ATR_GND_CTRL = true;
      PACE_CHARGE_CTRL = true;
      state = 1;
    state Sensing_Charge_C22_AAI
      entry:
      FRONTEND_CTRL = true;
      %Charge C22
      ATR_PACE_CTRL = false;
      VENT_PACE_CTRL = false;
      PACING_REF_PWM = (AAmplitude/5)*100;
      PACE_CHARGE_CTRL = true;
      state = 2;
      prev_state = 1;
    state Discharge_C22_ATR_AAI
      entry:
      FRONTEND_CTRL = false;
      PACE_CHARGE_CTRL = false;
      PACE_GND_CTRL = true;
      VENT_PACE_CTRL = false;
      ATR_GND_CTRL = false;
      Z_ATR_CTRL = false;
      Z_VENT_CTRL = false;
      VENT_GND_CTRL = false;
      ATR_PACE_CTRL = true;
      state =3;
      prev_state = 2;
    Sensing_Charge_C22_AAI -> Wait_AAI [order 1] : [ATR_CMP_DETECT == true]{natural = true}
    Wait_AAI -> Sensing_Charge_C22_AAI : [after(ARP, msec)]
    Discharge_C22_ATR_AAI -> Wait_AAI : [after(width,msec)]
    Sensing_Charge_C22_AAI -> Discharge_C22_ATR_AAI [order 2] : [after(LRI-ARP-width,msec) & ATR_CMP_DETECT == false & natural == false]
    Sensing_Charge_C22_AAI -> Discharge_C22_ATR_AAI [order 3] : [after(LRI-ARP,msec) & ATR_CMP_DETECT == false & natural == true]{natural = false}
  Mode_Selector -> Charge_C22_VOO [order 1] : [mode == 1]
  Mode_Selector -> Wait_VVI [order 2] : [mode == 2]
  (default) -> Mode_Selector
  Mode_Selector -> Charge_C22_AOO [order 3] : [mode == 3]
  Mode_Selector -> Wait_AAI [order 4] : [mode == 4]
  data: ATR_PACE_CTRL output boolean; VENT_PACE_CTRL output boolean; PACING_REF_PWM output double; PACE_CHARGE_CTRL output boolean; PACE_GND_CTRL output boolean; ATR_GND_CTRL output boolean; Z_ATR_CTRL output boolean; Z_VENT_CTRL output boolean; VENT_GND_CTRL output boolean; FRONTEND_CTRL output boolean; VENT_CMP_REF_PWM output double; VENT_CMP_DETECT input boolean; width input int16; URI input double; LRI input double; VRP input double [150..500]; ARP input double [150..500]; ATR_CMP_DETECT input boolean; ATR_CMP_REF_PWM output int16; mode input int16; VAmplitude input double; AAmplitude input double; state output int16; natural local boolean; prev_state output int16
